simulink model "LUT_kidney_35"  (R2023b)
settings: Solver=FixedStepAuto  StartTime=0  StopTime=10.1  FixedStep=Timegap  RelTol=1e-3
model workspace (MAT data in the model file):
  T1_input = 1.34
(part 2 of 3)

== system LUT_kidney_35/If Action Subsystem6/If Action Subsystem1/If Action Subsystem6/If Action Subsystem4 ==
  In1 : Inport
  Action Port : ActionPort  ActionPortLabel=elseif( u1 >= 1.035)
  LUT 1.04RR : Lookup_n-D  NumberOfTableDimensions=1  BreakpointsForDimension1=[420.026;533.7792;625.1446;723.0482;821.1572;919.1987;1017.154;1115.036;1212.861;1310.64;1408.383;1506.097;1603.789;1701.461;1799.118;1896.76;1994.389]  Table=[400;500;600;700;800;900;1000;1100;1200;1300;1400;1500;1600;1700;1800;1900;2000]  InternalRulePriority=Speed  RndMeth=Simplest
  Out1 : Outport
  wires:
  In1/1 -> LUT 1.04RR/1
  LUT 1.04RR/1 -> Out1/1

== system LUT_kidney_35/If Action Subsystem6/If Action Subsystem1/If Action Subsystem6/If Action Subsystem5 ==
  In1 : Inport
  Action Port : ActionPort  ActionPortLabel=elseif( u1 >= 1.055)
  LUT 1.06RR : Lookup_n-D  NumberOfTableDimensions=1  BreakpointsForDimension1=[419.5192;532.953;624.0409;721.6063;819.3558;917.0247;1014.599;1112.093;1209.526;1306.909;1404.254;1501.569;1598.859;1696.128;1793.38;1890.617;1987.841]  Table=[400;500;600;700;800;900;1000;1100;1200;1300;1400;1500;1600;1700;1800;1900;2000]  InternalRulePriority=Speed  RndMeth=Simplest
  Out1 : Outport
  wires:
  In1/1 -> LUT 1.06RR/1
  LUT 1.06RR/1 -> Out1/1

== system LUT_kidney_35/If Action Subsystem6/If Action Subsystem1/If Action Subsystem6/If Action Subsystem6 ==
  In1 : Inport
  Action Port : ActionPort  ActionPortLabel=elseif( u1 >= 1.045)
  LUT 1.05RR : Lookup_n-D  NumberOfTableDimensions=1  BreakpointsForDimension1=[419.7703;533.3612;624.5658;722.3181;820.245;918.098;1015.86;1113.547;1211.173;1308.752;1406.294;1503.806;1601.294;1698.763;1796.215;1893.652;1991.077]  Table=[400;500;600;700;800;900;1000;1100;1200;1300;1400;1500;1600;1700;1800;1900;2000]  InternalRulePriority=Speed  RndMeth=Simplest
  Out1 : Outport
  wires:
  In1/1 -> LUT 1.05RR/1
  LUT 1.05RR/1 -> Out1/1

== system LUT_kidney_35/If Action Subsystem6/If Action Subsystem1/If Action Subsystem6/If Action Subsystem7 ==
  In1 : Inport
  Action Port : ActionPort  ActionPortLabel=elseif( u1 >= 1.065)
  LUT 1.07RR : Lookup_n-D  NumberOfTableDimensions=1  BreakpointsForDimension1=[419.2724;532.5542;623.5094;720.9123;818.4888;915.9781;1013.368;1110.676;1207.919;1305.111;1402.264;1499.385;1596.48;1693.555;1790.611;1887.653;1984.68]  Table=[400;500;600;700;800;900;1000;1100;1200;1300;1400;1500;1600;1700;1800;1900;2000]  InternalRulePriority=Speed  RndMeth=Simplest
  Out1 : Outport
  wires:
  In1/1 -> LUT 1.07RR/1
  LUT 1.07RR/1 -> Out1/1

== system LUT_kidney_35/If Action Subsystem6/If Action Subsystem1/If Action Subsystem6/If Action Subsystem8 ==
  In1 : Inport
  Action Port : ActionPort  ActionPortLabel=elseif(u1 >= 1.075)
  LUT 1.08RR : Lookup_n-D  NumberOfTableDimensions=1  BreakpointsForDimension1=[419.0299;532.1644;622.9907;720.2354;817.6431;914.9571;1012.167;1109.292;1206.35;1303.355;1400.32;1497.252;1594.157;1691.041;1787.906;1884.756;1981.592]  Table=[400;500;600;700;800;900;1000;1100;1200;1300;1400;1500;1600;1700;1800;1900;2000]  InternalRulePriority=Speed  RndMeth=Simplest
  Out1 : Outport
  wires:
  In1/1 -> LUT 1.08RR/1
  LUT 1.08RR/1 -> Out1/1

== system LUT_kidney_35/If Action Subsystem6/If Action Subsystem1/If Action Subsystem6/If Action Subsystem9 ==
  In1 : Inport
  Action Port : ActionPort  ActionPortLabel=if(u1 >= 1.085)
  LUT 1.09RR : Lookup_n-D  NumberOfTableDimensions=1  BreakpointsForDimension1=[418.7915;531.7834;622.4844;719.5751;816.8181;913.9608;1010.995;1107.941;1204.818;1301.641;1398.421;1495.168;1591.887;1688.584;1785.262;1881.925;1978.573]  Table=[400;500;600;700;800;900;1000;1100;1200;1300;1400;1500;1600;1700;1800;1900;2000]  InternalRulePriority=Speed  RndMeth=Simplest
  Out1 : Outport
  wires:
  In1/1 -> LUT 1.09RR/1
  LUT 1.09RR/1 -> Out1/1

== system LUT_kidney_35/If Action Subsystem6/If Action Subsystem1/If Action Subsystem7/If Action Subsystem1 ==
  In1 : Inport
  Action Port : ActionPort  ActionPortLabel=elseif( u1 >= 1.215)
  LUT 1.22RR : Lookup_n-D  NumberOfTableDimensions=1  BreakpointsForDimension1=[416.0084;527.5016;616.8602;712.2688;807.6951;902.9352;998.0083;1092.951;1187.794;1282.56;1377.266;1471.925;1566.545;1661.135;1755.698;1850.24;1944.764]  Table=[400;500;600;700;800;900;1000;1100;1200;1300;1400;1500;1600;1700;1800;1900;2000]  InternalRulePriority=Speed  RndMeth=Simplest
  Out1 : Outport
  wires:
  In1/1 -> LUT 1.22RR/1
  LUT 1.22RR/1 -> Out1/1

== system LUT_kidney_35/If Action Subsystem6/If Action Subsystem1/If Action Subsystem7/If Action Subsystem10 ==
  In1 : Inport
  Action Port : ActionPort  ActionPortLabel=elseif( u1 >= 1.205)
  LUT 1.21RR : Lookup_n-D  NumberOfTableDimensions=1  BreakpointsForDimension1=[416.2043;527.7926;617.2379;712.7574;808.3047;903.6723;998.8776;1093.956;1188.937;1283.842;1378.69;1473.49;1568.254;1662.987;1757.695;1852.381;1947.05]  Table=[400;500;600;700;800;900;1000;1100;1200;1300;1400;1500;1600;1700;1800;1900;2000]  InternalRulePriority=Speed  RndMeth=Simplest
  Out1 : Outport
  wires:
  In1/1 -> LUT 1.21RR/1
  LUT 1.21RR/1 -> Out1/1

== system LUT_kidney_35/If Action Subsystem6/If Action Subsystem1/If Action Subsystem7/If Action Subsystem2 ==
  In1 : Inport
  Action Port : ActionPort  ActionPortLabel=else
  LUT 1.20RR : Lookup_n-D  NumberOfTableDimensions=1  BreakpointsForDimension1=[416.403;528.0893;617.6239;713.2569;808.928;904.426;999.7663;1094.983;1190.104;1285.152;1380.143;1475.089;1569.998;1664.878;1759.732;1854.566;1949.383]  Table=[400;500;600;700;800;900;1000;1100;1200;1300;1400;1500;1600;1700;1800;1900;2000]  InternalRulePriority=Speed  RndMeth=Simplest
  Out1 : Outport
  wires:
  In1/1 -> LUT 1.20RR/1
  LUT 1.20RR/1 -> Out1/1

== system LUT_kidney_35/If Action Subsystem6/If Action Subsystem1/If Action Subsystem7/If Action Subsystem3 ==
  In1 : Inport
  Action Port : ActionPort  ActionPortLabel=elseif( u1 >= 1.225)
  LUT 1.23RR : Lookup_n-D  NumberOfTableDimensions=1  BreakpointsForDimension1=[415.8151;527.216;616.4903;711.7908;807.0989;902.2141;997.1578;1091.968;1186.676;1281.305;1375.873;1470.392;1564.872;1659.32;1753.742;1848.142;1942.523]  Table=[400;500;600;700;800;900;1000;1100;1200;1300;1400;1500;1600;1700;1800;1900;2000]  InternalRulePriority=Speed  RndMeth=Simplest
  Out1 : Outport
  wires:
  In1/1 -> LUT 1.23RR/1
  LUT 1.23RR/1 -> Out1/1

== system LUT_kidney_35/If Action Subsystem6/If Action Subsystem1/If Action Subsystem7/If Action Subsystem4 ==
  In1 : Inport
  Action Port : ActionPort  ActionPortLabel=elseif( u1 >= 1.235)
  LUT 1.24RR : Lookup_n-D  NumberOfTableDimensions=1  BreakpointsForDimension1=[415.6243;526.9358;616.128;711.3231;806.5156;901.5086;996.3255;1091.006;1185.581;1280.076;1374.508;1468.89;1563.233;1657.543;1751.826;1846.086;1940.327]  Table=[400;500;600;700;800;900;1000;1100;1200;1300;1400;1500;1600;1700;1800;1900;2000]  InternalRulePriority=Speed  RndMeth=Simplest
  Out1 : Outport
  wires:
  In1/1 -> LUT 1.24RR/1
  LUT 1.24RR/1 -> Out1/1

== system LUT_kidney_35/If Action Subsystem6/If Action Subsystem1/If Action Subsystem7/If Action Subsystem5 ==
  In1 : Inport
  Action Port : ActionPort  ActionPortLabel=elseif( u1 >= 1.255)
  LUT 1.26RR : Lookup_n-D  NumberOfTableDimensions=1  BreakpointsForDimension1=[415.2502;526.3909;615.4257;710.4174;805.3864;900.1427;994.7137;1089.141;1183.459;1277.693;1371.861;1465.978;1560.052;1654.093;1748.106;1842.095;1936.064]  Table=[400;500;600;700;800;900;1000;1100;1200;1300;1400;1500;1600;1700;1800;1900;2000]  InternalRulePriority=Speed  RndMeth=Simplest
  Out1 : Outport
  wires:
  In1/1 -> LUT 1.26RR/1
  LUT 1.26RR/1 -> Out1/1

== system LUT_kidney_35/If Action Subsystem6/If Action Subsystem1/If Action Subsystem7/If Action Subsystem6 ==
  In1 : Inport
  Action Port : ActionPort  ActionPortLabel=elseif( u1 >= 1.245)
  LUT 1.25RR : Lookup_n-D  NumberOfTableDimensions=1  BreakpointsForDimension1=[415.4361;526.6608;615.7732;710.8654;805.9449;900.8182;995.511;1090.064;1184.509;1278.872;1373.171;1467.419;1561.626;1655.8;1749.947;1844.071;1938.175]  Table=[400;500;600;700;800;900;1000;1100;1200;1300;1400;1500;1600;1700;1800;1900;2000]  InternalRulePriority=Speed  RndMeth=Simplest
  Out1 : Outport
  wires:
  In1/1 -> LUT 1.25RR/1
  LUT 1.25RR/1 -> Out1/1

== system LUT_kidney_35/If Action Subsystem6/If Action Subsystem1/If Action Subsystem7/If Action Subsystem7 ==
  In1 : Inport
  Action Port : ActionPort  ActionPortLabel=elseif( u1 >= 1.265)
  LUT 1.27RR : Lookup_n-D  NumberOfTableDimensions=1  BreakpointsForDimension1=[415.0668;526.1258;615.0852;709.9789;804.8399;899.4815;993.9333;1088.238;1182.431;1276.538;1370.578;1464.565;1558.51;1652.42;1746.301;1840.158;1933.995]  Table=[400;500;600;700;800;900;1000;1100;1200;1300;1400;1500;1600;1700;1800;1900;2000]  InternalRulePriority=Speed  RndMeth=Simplest
  Out1 : Outport
  wires:
  In1/1 -> LUT 1.27RR/1
  LUT 1.27RR/1 -> Out1/1

== system LUT_kidney_35/If Action Subsystem6/If Action Subsystem1/If Action Subsystem7/If Action Subsystem8 ==
  In1 : Inport
  Action Port : ActionPort  ActionPortLabel=elseif(u1 >= 1.275)
  LUT 1.28RR : Lookup_n-D  NumberOfTableDimensions=1  BreakpointsForDimension1=[414.8856;525.8655;614.7515;709.5496;804.3049;898.8344;993.1693;1087.354;1181.425;1275.407;1369.321;1463.181;1556.998;1650.779;1744.531;1838.259;1931.966]  Table=[400;500;600;700;800;900;1000;1100;1200;1300;1400;1500;1600;1700;1800;1900;2000]  InternalRulePriority=Speed  RndMeth=Simplest
  Out1 : Outport
  wires:
  In1/1 -> LUT 1.28RR/1
  LUT 1.28RR/1 -> Out1/1

== system LUT_kidney_35/If Action Subsystem6/If Action Subsystem1/If Action Subsystem7/If Action Subsystem9 ==
  In1 : Inport
  Action Port : ActionPort  ActionPortLabel=if(u1 >= 1.285)
  LUT 1.29RR : Lookup_n-D  NumberOfTableDimensions=1  BreakpointsForDimension1=[414.7067;525.6098;614.4245;709.1292;803.7813;898.2008;992.4213;1086.488;1180.439;1274.299;1368.089;1461.825;1555.516;1649.171;1742.796;1836.396;1929.975]  Table=[400;500;600;700;800;900;1000;1100;1200;1300;1400;1500;1600;1700;1800;1900;2000]  InternalRulePriority=Speed  RndMeth=Simplest
  Out1 : Outport
  wires:
  In1/1 -> LUT 1.29RR/1
  LUT 1.29RR/1 -> Out1/1

== system LUT_kidney_35/If Action Subsystem6/If Action Subsystem1/If Action Subsystem8/If Action Subsystem1 ==
  In1 : Inport
  Action Port : ActionPort  ActionPortLabel=elseif( u1 >= 1.315)
  LUT 1.32RR : Lookup_n-D  NumberOfTableDimensions=1  BreakpointsForDimension1=[414.1829;524.8694;613.4816;707.9195;802.2751;896.3784;990.2688;1083.996;1177.598;1271.106;1364.539;1457.913;1551.24;1644.53;1737.787;1831.019;1924.228]  Table=[400;500;600;700;800;900;1000;1100;1200;1300;1400;1500;1600;1700;1800;1900;2000]  InternalRulePriority=Speed  RndMeth=Simplest
  Out1 : Outport
  wires:
  In1/1 -> LUT 1.32RR/1
  LUT 1.32RR/1 -> Out1/1

== system LUT_kidney_35/If Action Subsystem6/If Action Subsystem1/If Action Subsystem8/If Action Subsystem10 ==
  In1 : Inport
  Action Port : ActionPort  ActionPortLabel=elseif( u1 >= 1.305)
  LUT 1.31RR : Lookup_n-D  NumberOfTableDimensions=1  BreakpointsForDimension1=[414.3554;525.1119;613.7897;708.3144;802.7666;896.9732;990.9714;1084.81;1178.526;1272.149;1365.699;1459.191;1552.638;1646.047;1739.425;1832.777;1926.107]  Table=[400;500;600;700;800;900;1000;1100;1200;1300;1400;1500;1600;1700;1800;1900;2000]  InternalRulePriority=Speed  RndMeth=Simplest
  Out1 : Outport
  wires:
  In1/1 -> LUT 1.31RR/1
  LUT 1.31RR/1 -> Out1/1

== system LUT_kidney_35/If Action Subsystem6/If Action Subsystem1/If Action Subsystem8/If Action Subsystem2 ==
  In1 : Inport
  Action Port : ActionPort  ActionPortLabel=else
  LUT 1.30RR : Lookup_n-D  NumberOfTableDimensions=1  BreakpointsForDimension1=[414.53;525.3587;614.1039;708.7176;803.2686;897.5805;991.6888;1085.64;1179.472;1273.213;1366.882;1460.495;1554.063;1647.593;1741.094;1834.569;1928.023]  Table=[400;500;600;700;800;900;1000;1100;1200;1300;1400;1500;1600;1700;1800;1900;2000]  InternalRulePriority=Speed  RndMeth=Simplest
  Out1 : Outport
  wires:
  In1/1 -> LUT 1.30RR/1
  LUT 1.30RR/1 -> Out1/1

== system LUT_kidney_35/If Action Subsystem6/If Action Subsystem1/If Action Subsystem8/If Action Subsystem3 ==
  In1 : Inport
  Action Port : ActionPort  ActionPortLabel=elseif( u1 >= 1.325)
  LUT 1.33RR : Lookup_n-D  NumberOfTableDimensions=1  BreakpointsForDimension1=[414.0125;524.6311;613.1794;707.5326;801.7937;895.7959;989.5805;1083.198;1176.689;1270.083;1363.401;1456.66;1549.87;1643.041;1736.181;1829.293;1922.383]  Table=[400;500;600;700;800;900;1000;1100;1200;1300;1400;1500;1600;1700;1800;1900;2000]  InternalRulePriority=Speed  RndMeth=Simplest
  Out1 : Outport
  wires:
  In1/1 -> LUT 1.33RR/1
  LUT 1.33RR/1 -> Out1/1

== system LUT_kidney_35/If Action Subsystem6/If Action Subsystem1/If Action Subsystem8/If Action Subsystem4 ==
  In1 : Inport
  Action Port : ActionPort  ActionPortLabel=elseif( u1 >= 1.335)
  LUT 1.34RR : Lookup_n-D  NumberOfTableDimensions=1  BreakpointsForDimension1=[413.8441;524.3968;612.8831;707.1536;801.3223;895.2254;988.9063;1082.417;1175.799;1269.081;1362.286;1455.431;1548.526;1641.582;1734.605;1827.601;1920.573]  Table=[400;500;600;700;800;900;1000;1100;1200;1300;1400;1500;1600;1700;1800;1900;2000]  InternalRulePriority=Speed  RndMeth=Simplest
  Out1 : Outport
  wires:
  In1/1 -> LUT 1.34RR/1
  LUT 1.34RR/1 -> Out1/1

== system LUT_kidney_35/If Action Subsystem6/If Action Subsystem1/If Action Subsystem8/If Action Subsystem5 ==
  In1 : Inport
  Action Port : ActionPort  ActionPortLabel=elseif( u1 >= 1.355)
  LUT 1.36RR : Lookup_n-D  NumberOfTableDimensions=1  BreakpointsForDimension1=[413.5131;523.94;612.3074;706.4184;800.4081;894.1191;987.5986;1080.901;1174.07;1267.135;1360.12;1453.043;1545.914;1638.744;1731.541;1824.309;1917.053]  Table=[400;500;600;700;800;900;1000;1100;1200;1300;1400;1500;1600;1700;1800;1900;2000]  InternalRulePriority=Speed  RndMeth=Simplest
  Out1 : Outport
  wires:
  In1/1 -> LUT 1.36RR/1
  LUT 1.36RR/1 -> Out1/1

== system LUT_kidney_35/If Action Subsystem6/If Action Subsystem1/If Action Subsystem8/If Action Subsystem6 ==
  In1 : Inport
  Action Port : ActionPort  ActionPortLabel=elseif( u1 >= 1.345)
  LUT 1.35RR : Lookup_n-D  NumberOfTableDimensions=1  BreakpointsForDimension1=[413.6776;524.1665;612.5925;706.7823;800.8605;894.6666;988.2458;1081.652;1174.926;1268.098;1361.193;1454.225;1547.207;1640.149;1733.058;1825.939;1918.797]  Table=[400;500;600;700;800;900;1000;1100;1200;1300;1400;1500;1600;1700;1800;1900;2000]  InternalRulePriority=Speed  RndMeth=Simplest
  Out1 : Outport
  wires:
  In1/1 -> LUT 1.35RR/1
  LUT 1.35RR/1 -> Out1/1

== system LUT_kidney_35/If Action Subsystem6/If Action Subsystem1/If Action Subsystem8/If Action Subsystem7 ==
  In1 : Inport
  Action Port : ActionPort  ActionPortLabel=elseif( u1 >= 1.365)
  LUT 1.37RR : Lookup_n-D  NumberOfTableDimensions=1  BreakpointsForDimension1=[413.3504;523.7173;612.0277;706.0618;799.9648;893.5827;986.9645;1080.166;1173.231;1266.19;1359.069;1451.883;1544.645;1637.365;1730.051;1822.708;1915.341]  Table=[400;500;600;700;800;900;1000;1100;1200;1300;1400;1500;1600;1700;1800;1900;2000]  InternalRulePriority=Speed  RndMeth=Simplest
  Out1 : Outport
  wires:
  In1/1 -> LUT 1.37RR/1
  LUT 1.37RR/1 -> Out1/1

== system LUT_kidney_35/If Action Subsystem6/If Action Subsystem1/If Action Subsystem8/If Action Subsystem8 ==
  In1 : Inport
  Action Port : ActionPort  ActionPortLabel=elseif(u1 >= 1.375)
  LUT 1.38RR : Lookup_n-D  NumberOfTableDimensions=1  BreakpointsForDimension1=[413.1896;523.4982;611.7533;705.7122;799.5306;893.0572;986.343;1079.445;1172.408;1265.264;1358.037;1450.745;1543.399;1636.012;1728.589;1821.137;1913.66]  Table=[400;500;600;700;800;900;1000;1100;1200;1300;1400;1500;1600;1700;1800;1900;2000]  InternalRulePriority=Speed  RndMeth=Simplest
  Out1 : Outport
  wires:
  In1/1 -> LUT 1.38RR/1
  LUT 1.38RR/1 -> Out1/1

== system LUT_kidney_35/If Action Subsystem6/If Action Subsystem1/If Action Subsystem8/If Action Subsystem9 ==
  In1 : Inport
  Action Port : ActionPort  ActionPortLabel=if(u1 >= 1.385)
  LUT 1.39RR : Lookup_n-D  NumberOfTableDimensions=1  BreakpointsForDimension1=[413.0306;523.2827;611.4839;705.3696;799.1051;892.5422;985.7339;1078.739;1171.601;1264.356;1357.025;1449.628;1542.177;1634.683;1727.154;1819.594;1912.01]  Table=[400;500;600;700;800;900;1000;1100;1200;1300;1400;1500;1600;1700;1800;1900;2000]  InternalRulePriority=Speed  RndMeth=Simplest
  Out1 : Outport
  wires:
  In1/1 -> LUT 1.39RR/1
  LUT 1.39RR/1 -> Out1/1

== system LUT_kidney_35/If Action Subsystem6/If Action Subsystem1/If Action Subsystem9/If Action Subsystem1 ==
  In1 : Inport
  Action Port : ActionPort  ActionPortLabel=elseif( u1 >= 1.415)
  LUT 1.42RR : Lookup_n-D  NumberOfTableDimensions=1  BreakpointsForDimension1=[412.5639;522.6569;610.7055;704.3815;797.8789;891.0583;983.9782;1076.701;1169.274;1261.733;1354.103;1446.402;1538.645;1630.843;1723.003;1815.131;1907.234]  Table=[400;500;600;700;800;900;1000;1100;1200;1300;1400;1500;1600;1700;1800;1900;2000]  InternalRulePriority=Speed  RndMeth=Simplest
  Out1 : Outport
  wires:
  In1/1 -> LUT 1.42RR/1
  LUT 1.42RR/1 -> Out1/1

== system LUT_kidney_35/If Action Subsystem6/If Action Subsystem1/If Action Subsystem9/If Action Subsystem10 ==
  In1 : Inport
  Action Port : ActionPort  ActionPortLabel=elseif( u1 >= 1.405)
  LUT 1.41RR : Lookup_n-D  NumberOfTableDimensions=1  BreakpointsForDimension1=[412.7178;522.8621;610.9602;704.7044;798.2794;891.543;984.5518;1077.367;1170.035;1262.59;1355.058;1447.457;1539.801;1632.099;1724.361;1816.592;1908.797]  Table=[400;500;600;700;800;900;1000;1100;1200;1300;1400;1500;1600;1700;1800;1900;2000]  InternalRulePriority=Speed  RndMeth=Simplest
  Out1 : Outport
  wires:
  In1/1 -> LUT 1.41RR/1
  LUT 1.41RR/1 -> Out1/1

== system LUT_kidney_35/If Action Subsystem6/If Action Subsystem1/If Action Subsystem9/If Action Subsystem2 ==
  In1 : Inport
  Action Port : ActionPort  ActionPortLabel=else
  LUT 1.40RR : Lookup_n-D  NumberOfTableDimensions=1  BreakpointsForDimension1=[412.8733;523.0707;611.2196;705.0337;798.6881;892.0376;985.137;1078.046;1170.81;1263.464;1356.032;1448.532;1540.978;1633.38;1725.745;1818.08;1910.389]  Table=[400;500;600;700;800;900;1000;1100;1200;1300;1400;1500;1600;1700;1800;1900;2000]  InternalRulePriority=Speed  RndMeth=Simplest
  Out1 : Outport
  wires:
  In1/1 -> LUT 1.40RR/1
  LUT 1.40RR/1 -> Out1/1

== system LUT_kidney_35/If Action Subsystem6/If Action Subsystem1/If Action Subsystem9/If Action Subsystem3 ==
  In1 : Inport
  Action Port : ActionPort  ActionPortLabel=elseif( u1 >= 1.425)
  LUT 1.43RR : Lookup_n-D  NumberOfTableDimensions=1  BreakpointsForDimension1=[412.4118;522.4548;610.4555;704.0649;797.4863;890.5831;983.4159;1076.048;1168.528;1260.892;1353.165;1445.366;1537.511;1629.609;1721.669;1813.697;1905.698]  Table=[400;500;600;700;800;900;1000;1100;1200;1300;1400;1500;1600;1700;1800;1900;2000]  InternalRulePriority=Speed  RndMeth=Simplest
  Out1 : Outport
  wires:
  In1/1 -> LUT 1.43RR/1
  LUT 1.43RR/1 -> Out1/1

== system LUT_kidney_35/If Action Subsystem6/If Action Subsystem1/If Action Subsystem9/If Action Subsystem4 ==
  In1 : Inport
  Action Port : ActionPort  ActionPortLabel=elseif( u1 >= 1.435)
  LUT 1.44RR : Lookup_n-D  NumberOfTableDimensions=1  BreakpointsForDimension1=[412.2612;522.256;610.21;703.7545;797.1014;890.1174;982.8646;1075.408;1167.796;1260.066;1352.244;1444.35;1536.397;1628.397;1720.359;1812.288;1904.189]  Table=[400;500;600;700;800;900;1000;1100;1200;1300;1400;1500;1600;1700;1800;1900;2000]  InternalRulePriority=Speed  RndMeth=Simplest
  Out1 : Outport
  wires:
  In1/1 -> LUT 1.44RR/1
  LUT 1.44RR/1 -> Out1/1

== system LUT_kidney_35/If Action Subsystem6/If Action Subsystem1/If Action Subsystem9/If Action Subsystem5 ==
  In1 : Inport
  Action Port : ActionPort  ActionPortLabel=elseif( u1 >= 1.455)
  LUT 1.46RR : Lookup_n-D  NumberOfTableDimensions=1  BreakpointsForDimension1=[411.965;521.8675;609.7322;703.1513;796.3542;889.2132;981.794;1074.164;1166.374;1258.462;1350.455;1442.372;1534.23;1626.039;1717.808;1809.543;1901.251]  Table=[400;500;600;700;800;900;1000;1100;1200;1300;1400;1500;1600;1700;1800;1900;2000]  InternalRulePriority=Speed  RndMeth=Simplest
  Out1 : Outport
  wires:
  In1/1 -> LUT 1.46RR/1
  LUT 1.46RR/1 -> Out1/1

== system LUT_kidney_35/If Action Subsystem6/If Action Subsystem1/If Action Subsystem9/If Action Subsystem6 ==
  In1 : Inport
  Action Port : ActionPort  ActionPortLabel=elseif( u1 >= 1.445)
  LUT 1.45RR : Lookup_n-D  NumberOfTableDimensions=1  BreakpointsForDimension1=[412.1123;522.0602;609.9689;703.45;796.7241;889.6608;982.324;1074.78;1167.078;1259.256;1351.341;1443.352;1535.304;1627.207;1719.072;1810.903;1902.707]  Table=[400;500;600;700;800;900;1000;1100;1200;1300;1400;1500;1600;1700;1800;1900;2000]  InternalRulePriority=Speed  RndMeth=Simplest
  Out1 : Outport
  wires:
  In1/1 -> LUT 1.45RR/1
  LUT 1.45RR/1 -> Out1/1

== system LUT_kidney_35/If Action Subsystem6/If Action Subsystem1/If Action Subsystem9/If Action Subsystem7 ==
  In1 : Inport
  Action Port : ActionPort  ActionPortLabel=elseif( u1 >= 1.465)
  LUT 1.47RR : Lookup_n-D  NumberOfTableDimensions=1  BreakpointsForDimension1=[411.8192;521.6777;609.4996;702.8584;795.9916;888.7743;981.2742;1073.56;1165.683;1257.682;1349.584;1441.411;1533.176;1624.891;1716.566;1808.207;1899.82]  Table=[400;500;600;700;800;900;1000;1100;1200;1300;1400;1500;1600;1700;1800;1900;2000]  InternalRulePriority=Speed  RndMeth=Simplest
  Out1 : Outport
  wires:
  In1/1 -> LUT 1.47RR/1
  LUT 1.47RR/1 -> Out1/1

== system LUT_kidney_35/If Action Subsystem6/If Action Subsystem1/If Action Subsystem9/If Action Subsystem8 ==
  In1 : Inport
  Action Port : ActionPort  ActionPortLabel=elseif(u1 >= 1.475)
  LUT 1.48RR : Lookup_n-D  NumberOfTableDimensions=1  BreakpointsForDimension1=[411.6749;521.4908;609.2713;702.571;795.636;888.344;980.7645;1072.967;1165.005;1256.917;1348.73;1440.466;1532.14;1623.764;1715.346;1806.894;1898.413]  Table=[400;500;600;700;800;900;1000;1100;1200;1300;1400;1500;1600;1700;1800;1900;2000]  InternalRulePriority=Speed  RndMeth=Simplest
  Out1 : Outport
  wires:
  In1/1 -> LUT 1.48RR/1
  LUT 1.48RR/1 -> Out1/1

== system LUT_kidney_35/If Action Subsystem6/If Action Subsystem1/If Action Subsystem9/If Action Subsystem9 ==
  In1 : Inport
  Action Port : ActionPort  ActionPortLabel=if(u1 >= 1.485)
  LUT 1.49RR : Lookup_n-D  NumberOfTableDimensions=1  BreakpointsForDimension1=[411.5321;521.3067;609.0469;702.2891;795.2873;887.922;980.2646;1072.386;1164.34;1256.165;1347.891;1439.539;1531.123;1622.656;1714.148;1805.604;1897.031]  Table=[400;500;600;700;800;900;1000;1100;1200;1300;1400;1500;1600;1700;1800;1900;2000]  InternalRulePriority=Speed  RndMeth=Simplest
  Out1 : Outport
  wires:
  In1/1 -> LUT 1.49RR/1
  LUT 1.49RR/1 -> Out1/1

== system LUT_kidney_35/If Action Subsystem6/If Action Subsystem2/If Action Subsystem5/If Action Subsystem1 ==
  In1 : Inport
  Action Port : ActionPort  ActionPortLabel=elseif( u1 >= 1.615)
  LUT 1.62RR : Lookup_n-D  NumberOfTableDimensions=1  BreakpointsForDimension1=[409.8015;519.1447;606.459;699.0681;791.3171;883.1195;974.569;1065.752;1156.734;1247.561;1338.268;1428.88;1519.417;1609.892;1700.316;1790.698;1881.045]  Table=[400;500;600;700;800;900;1000;1100;1200;1300;1400;1500;1600;1700;1800;1900;2000]  InternalRulePriority=Speed  RndMeth=Simplest
  Out1 : Outport
  wires:
  In1/1 -> LUT 1.62RR/1
  LUT 1.62RR/1 -> Out1/1

== system LUT_kidney_35/If Action Subsystem6/If Action Subsystem2/If Action Subsystem5/If Action Subsystem10 ==
  In1 : Inport
  Action Port : ActionPort  ActionPortLabel=elseif( u1>= 1.605)
  LUT 1.61RR : Lookup_n-D  NumberOfTableDimensions=1  BreakpointsForDimension1=[409.9269;519.2971;606.6384;699.2892;791.5887;883.4479;974.9589;1066.207;1157.256;1248.153;1338.931;1429.616;1520.226;1610.775;1701.275;1791.733;1882.156]  Table=[400;500;600;700;800;900;1000;1100;1200;1300;1400;1500;1600;1700;1800;1900;2000]  InternalRulePriority=Speed  RndMeth=Simplest
  Out1 : Outport
  wires:
  In1/1 -> LUT 1.61RR/1
  LUT 1.61RR/1 -> Out1/1

== system LUT_kidney_35/If Action Subsystem6/If Action Subsystem2/If Action Subsystem5/If Action Subsystem2 ==
  In1 : Inport
  Action Port : ActionPort  ActionPortLabel=else
  LUT 1.60RR : Lookup_n-D  NumberOfTableDimensions=1  BreakpointsForDimension1=[410.0535;519.4517;606.8208;699.5145;791.8656;883.7827;975.3562;1066.67;1157.788;1248.756;1339.606;1430.365;1521.05;1611.674;1702.25;1792.784;1883.285]  Table=[400;500;600;700;800;900;1000;1100;1200;1300;1400;1500;1600;1700;1800;1900;2000]  InternalRulePriority=Speed  RndMeth=Simplest
  Out1 : Outport
  wires:
  In1/1 -> LUT 1.60RR/1
  LUT 1.60RR/1 -> Out1/1

== system LUT_kidney_35/If Action Subsystem6/If Action Subsystem2/If Action Subsystem5/If Action Subsystem3 ==
  In1 : Inport
  Action Port : ActionPort  ActionPortLabel=elseif( u1 >= 1.625)
  LUT 1.63RR : Lookup_n-D  NumberOfTableDimensions=1  BreakpointsForDimension1=[409.6773;518.9944;606.2826;698.8509;791.0505;882.7972;974.1864;1065.306;1156.221;1246.979;1337.616;1428.157;1518.621;1609.023;1699.373;1789.681;1879.953]  Table=[400;500;600;700;800;900;1000;1100;1200;1300;1400;1500;1600;1700;1800;1900;2000]  InternalRulePriority=Speed  RndMeth=Simplest
  Out1 : Outport
  wires:
  In1/1 -> LUT 1.63RR/1
  LUT 1.63RR/1 -> Out1/1

== system LUT_kidney_35/If Action Subsystem6/If Action Subsystem2/If Action Subsystem5/If Action Subsystem4 ==
  In1 : Inport
  Action Port : ActionPort  ActionPortLabel=elseif( u1 >= 1.635)
  LUT 1.64RR : Lookup_n-D  NumberOfTableDimensions=1  BreakpointsForDimension1=[409.5542;518.8461;606.1091;698.6376;790.7889;882.4803;973.8109;1064.867;1155.717;1246.408;1336.976;1427.446;1517.839;1608.168;1698.446;1788.68;1878.879]  Table=[400;500;600;700;800;900;1000;1100;1200;1300;1400;1500;1600;1700;1800;1900;2000]  InternalRulePriority=Speed  RndMeth=Simplest
  Out1 : Outport
  wires:
  In1/1 -> LUT 1.64RR/1
  LUT 1.64RR/1 -> Out1/1

== system LUT_kidney_35/If Action Subsystem6/If Action Subsystem2/If Action Subsystem5/If Action Subsystem5 ==
  In1 : Inport
  Action Port : ActionPort  ActionPortLabel=elseif( u1 >= 1.655)
  LUT 1.66RR : Lookup_n-D  NumberOfTableDimensions=1  BreakpointsForDimension1=[409.3117;518.5555;605.7705;698.2225;790.2803;881.8663;973.0807;1064.015;1154.736;1245.296;1335.729;1426.061;1516.314;1606.502;1696.637;1786.728;1876.781]  Table=[400;500;600;700;800;900;1000;1100;1200;1300;1400;1500;1600;1700;1800;1900;2000]  InternalRulePriority=Speed  RndMeth=Simplest
  Out1 : Outport
  wires:
  In1/1 -> LUT 1.66RR/1
  LUT 1.66RR/1 -> Out1/1

== system LUT_kidney_35/If Action Subsystem6/If Action Subsystem2/If Action Subsystem5/If Action Subsystem6 ==
  In1 : Inport
  Action Port : ActionPort  ActionPortLabel=elseif( u1 >= 1.645)
  LUT 1.65RR : Lookup_n-D  NumberOfTableDimensions=1  BreakpointsForDimension1=[409.4324;518.6998;605.9384;698.4282;790.5322;882.1708;973.4424;1064.437;1155.222;1245.847;1336.347;1426.748;1517.07;1607.328;1697.534;1787.696;1877.821]  Table=[400;500;600;700;800;900;1000;1100;1200;1300;1400;1500;1600;1700;1800;1900;2000]  InternalRulePriority=Speed  RndMeth=Simplest
  Out1 : Outport
  wires:
  In1/1 -> LUT 1.65RR/1
  LUT 1.65RR/1 -> Out1/1

== system LUT_kidney_35/If Action Subsystem6/If Action Subsystem2/If Action Subsystem5/If Action Subsystem7 ==
  In1 : Inport
  Action Port : ActionPort  ActionPortLabel=elseif( u1 >= 1.665)
  LUT 1.67RR : Lookup_n-D  NumberOfTableDimensions=1  BreakpointsForDimension1=[409.1921;518.4132;605.6053;698.0205;790.033;881.5675;972.7257;1063.6;1154.259;1244.754;1335.121;1425.387;1515.571;1605.69;1695.755;1785.775;1875.758]  Table=[400;500;600;700;800;900;1000;1100;1200;1300;1400;1500;1600;1700;1800;1900;2000]  InternalRulePriority=Speed  RndMeth=Simplest
  Out1 : Outport
  wires:
  In1/1 -> LUT 1.67RR/1
  LUT 1.67RR/1 -> Out1/1

== system LUT_kidney_35/If Action Subsystem6/If Action Subsystem2/If Action Subsystem5/If Action Subsystem8 ==
  In1 : Inport
  Action Port : ActionPort  ActionPortLabel=elseif(u1 >= 1.675)
  LUT 1.68RR : Lookup_n-D  NumberOfTableDimensions=1  BreakpointsForDimension1=[409.0736;518.2727;605.4428;697.8221;789.7904;881.2743;972.3773;1063.193;1153.791;1244.222;1334.524;1424.723;1514.841;1604.891;1694.887;1784.838;1874.751]  Table=[400;500;600;700;800;900;1000;1100;1200;1300;1400;1500;1600;1700;1800;1900;2000]  InternalRulePriority=Speed  RndMeth=Simplest
  Out1 : Outport
  wires:
  In1/1 -> LUT 1.68RR/1
  LUT 1.68RR/1 -> Out1/1

== system LUT_kidney_35/If Action Subsystem6/If Action Subsystem2/If Action Subsystem5/If Action Subsystem9 ==
  In1 : Inport
  Action Port : ActionPort  ActionPortLabel=if(u1 >= 1.685)
  LUT 1.69RR : Lookup_n-D  NumberOfTableDimensions=1  BreakpointsForDimension1=[408.9562;518.1341;605.2828;697.6273;789.5522;880.9866;972.0354;1062.793;1153.331;1243.7;1333.938;1424.071;1514.122;1604.106;1694.034;1783.916;1873.759]  Table=[400;500;600;700;800;900;1000;1100;1200;1300;1400;1500;1600;1700;1800;1900;2000]  InternalRulePriority=Speed  RndMeth=Simplest
  Out1 : Outport
  wires:
  In1/1 -> LUT 1.69RR/1
  LUT 1.69RR/1 -> Out1/1

== system LUT_kidney_35/If Action Subsystem6/If Action Subsystem2/If Action Subsystem6/If Action Subsystem1 ==
  In1 : Inport
  Action Port : ActionPort  ActionPortLabel=elseif( u1 >= 1.515)
  LUT 1.52RR : Lookup_n-D  NumberOfTableDimensions=1  BreakpointsForDimension1=[411.1125;520.7708;608.3971;701.4748;794.281;886.7045;978.8217;1070.707;1162.418;1253.994;1345.466;1436.855;1528.179;1619.449;1710.676;1801.866;1893.025]  Table=[400;500;600;700;800;900;1000;1100;1200;1300;1400;1500;1600;1700;1800;1900;2000]  InternalRulePriority=Speed  RndMeth=Simplest
  Out1 : Outport
  wires:
  In1/1 -> LUT 1.52RR/1
  LUT 1.52RR/1 -> Out1/1

== system LUT_kidney_35/If Action Subsystem6/If Action Subsystem2/If Action Subsystem6/If Action Subsystem10 ==
  In1 : Inport
  Action Port : ActionPort  ActionPortLabel=elseif( u1 >= 1.505)
  LUT 1.51RR : Lookup_n-D  NumberOfTableDimensions=1  BreakpointsForDimension1=[411.2509;520.9468;608.6099;701.7411;794.6099;887.1024;979.2934;1071.256;1163.046;1254.704;1346.26;1437.734;1529.143;1620.5;1711.813;1803.09;1894.337]  Table=[400;500;600;700;800;900;1000;1100;1200;1300;1400;1500;1600;1700;1800;1900;2000]  InternalRulePriority=Speed  RndMeth=Simplest
  Out1 : Outport
  wires:
  In1/1 -> LUT 1.51RR/1
  LUT 1.51RR/1 -> Out1/1

== system LUT_kidney_35/If Action Subsystem6/If Action Subsystem2/If Action Subsystem6/If Action Subsystem2 ==
  In1 : Inport
  Action Port : ActionPort  ActionPortLabel=else
  LUT 1.50RR : Lookup_n-D  NumberOfTableDimensions=1  BreakpointsForDimension1=[411.3908;521.1254;608.8265;702.0125;794.9453;887.5082;979.7743;1071.816;1163.687;1255.428;1347.068;1438.628;1530.124;1621.568;1712.97;1804.336;1895.673]  Table=[400;500;600;700;800;900;1000;1100;1200;1300;1400;1500;1600;1700;1800;1900;2000]  InternalRulePriority=Speed  RndMeth=Simplest
  Out1 : Outport
  wires:
  In1/1 -> LUT 1.50RR/1
  LUT 1.50RR/1 -> Out1/1

== system LUT_kidney_35/If Action Subsystem6/If Action Subsystem2/If Action Subsystem6/If Action Subsystem3 ==
  In1 : Inport
  Action Port : ActionPort  ActionPortLabel=elseif( u1 >= 1.525)
  LUT 1.53RR : Lookup_n-D  NumberOfTableDimensions=1  BreakpointsForDimension1=[410.9755;520.5974;608.188;701.2134;793.9584;886.3141;978.359;1070.169;1161.801;1253.296;1344.686;1435.993;1527.232;1618.417;1709.558;1800.662;1891.734]  Table=[400;500;600;700;800;900;1000;1100;1200;1300;1400;1500;1600;1700;1800;1900;2000]  InternalRulePriority=Speed  RndMeth=Simplest
  Out1 : Outport
  wires:
  In1/1 -> LUT 1.53RR/1
  LUT 1.53RR/1 -> Out1/1

== system LUT_kidney_35/If Action Subsystem6/If Action Subsystem2/If Action Subsystem6/If Action Subsystem4 ==
  In1 : Inport
  Action Port : ActionPort  ActionPortLabel=elseif( u1 >= 1.535)
  LUT 1.54RR : Lookup_n-D  NumberOfTableDimensions=1  BreakpointsForDimension1=[410.8398;520.4266;607.9825;700.957;793.642;885.9313;977.9051;1069.64;1161.195;1252.612;1343.921;1435.145;1526.302;1617.403;1708.46;1799.478;1890.465]  Table=[400;500;600;700;800;900;1000;1100;1200;1300;1400;1500;1600;1700;1800;1900;2000]  InternalRulePriority=Speed  RndMeth=Simplest
  Out1 : Outport
  wires:
  In1/1 -> LUT 1.54RR/1
  LUT 1.54RR/1 -> Out1/1

== system LUT_kidney_35/If Action Subsystem6/If Action Subsystem2/If Action Subsystem6/If Action Subsystem5 ==
  In1 : Inport
  Action Port : ActionPort  ActionPortLabel=elseif( u1 >= 1.555)
  LUT 1.56RR : Lookup_n-D  NumberOfTableDimensions=1  BreakpointsForDimension1=[410.5725;520.0923;607.582;700.4582;793.027;885.1874;977.0229;1068.613;1160.017;1251.279;1342.431;1433.495;1524.49;1615.427;1706.319;1797.171;1887.991]  Table=[400;500;600;700;800;900;1000;1100;1200;1300;1400;1500;1600;1700;1800;1900;2000]  InternalRulePriority=Speed  RndMeth=Simplest
  Out1 : Outport
  wires:
  In1/1 -> LUT 1.56RR/1
  LUT 1.56RR/1 -> Out1/1

== system LUT_kidney_35/If Action Subsystem6/If Action Subsystem2/If Action Subsystem6/If Action Subsystem6 ==
  In1 : Inport
  Action Port : ActionPort  ActionPortLabel=elseif( u1 >= 1.545)
  LUT 1.55RR : Lookup_n-D  NumberOfTableDimensions=1  BreakpointsForDimension1=[410.7055;520.2582;607.7805;700.7053;793.3316;885.5558;977.4598;1069.122;1160.601;1251.939;1343.169;1434.313;1525.388;1616.407;1707.38;1798.315;1889.218]  Table=[400;500;600;700;800;900;1000;1100;1200;1300;1400;1500;1600;1700;1800;1900;2000]  InternalRulePriority=Speed  RndMeth=Simplest
  Out1 : Outport
  wires:
  In1/1 -> LUT 1.55RR/1
  LUT 1.55RR/1 -> Out1/1

== system LUT_kidney_35/If Action Subsystem6/If Action Subsystem2/If Action Subsystem6/If Action Subsystem7 ==
  In1 : Inport
  Action Port : ActionPort  ActionPortLabel=elseif( u1 >= 1.565)
  LUT 1.57RR : Lookup_n-D  NumberOfTableDimensions=1  BreakpointsForDimension1=[410.4408;519.9287;607.3868;700.2157;792.7283;884.8261;976.5943;1068.114;1159.444;1250.631;1341.706;1432.692;1523.607;1614.465;1705.275;1796.047;1886.785]  Table=[400;500;600;700;800;900;1000;1100;1200;1300;1400;1500;1600;1700;1800;1900;2000]  InternalRulePriority=Speed  RndMeth=Simplest
  Out1 : Outport
  wires:
  In1/1 -> LUT 1.57RR/1
  LUT 1.57RR/1 -> Out1/1

== system LUT_kidney_35/If Action Subsystem6/If Action Subsystem2/If Action Subsystem6/If Action Subsystem8 ==
  In1 : Inport
  Action Port : ActionPort  ActionPortLabel=elseif(u1 >= 1.575)
  LUT 1.58RR : Lookup_n-D  NumberOfTableDimensions=1  BreakpointsForDimension1=[410.3104;519.7674;607.195;699.9776;792.4352;884.4716;976.1738;1067.623;1158.882;1249.995;1340.993;1431.902;1522.74;1613.519;1704.25;1794.941;1885.599]  Table=[400;500;600;700;800;900;1000;1100;1200;1300;1400;1500;1600;1700;1800;1900;2000]  InternalRulePriority=Speed  RndMeth=Simplest
  Out1 : Outport
  wires:
  In1/1 -> LUT 1.58RR/1
  LUT 1.58RR/1 -> Out1/1

== system LUT_kidney_35/If Action Subsystem6/If Action Subsystem2/If Action Subsystem6/If Action Subsystem9 ==
  In1 : Inport
  Action Port : ActionPort  ActionPortLabel=if(u1 >= 1.585)
  LUT 1.59RR : Lookup_n-D  NumberOfTableDimensions=1  BreakpointsForDimension1=[410.1813;519.6085;607.0063;699.7439;792.1477;884.1239;975.7611;1067.142;1158.33;1249.37;1340.294;1431.127;1521.887;1612.588;1703.241;1793.854;1884.432]  Table=[400;500;600;700;800;900;1000;1100;1200;1300;1400;1500;1600;1700;1800;1900;2000]  InternalRulePriority=Speed  RndMeth=Simplest
  Out1 : Outport
  wires:
  In1/1 -> LUT 1.59RR/1
  LUT 1.59RR/1 -> Out1/1

== system LUT_kidney_35/If Action Subsystem6/If Action Subsystem2/If Action Subsystem7/If Action Subsystem1 ==
  In1 : Inport
  Action Port : ActionPort  ActionPortLabel=elseif( u1 >= 1.715)
  LUT 1.72RR : Lookup_n-D  NumberOfTableDimensions=1  BreakpointsForDimension1=[408.6106;517.7291;604.8183;697.0631;788.8636;880.155;971.0469;1061.637;1152;1242.187;1332.238;1422.181;1512.038;1601.825;1691.555;1781.237;1870.879]  Table=[400;500;600;700;800;900;1000;1100;1200;1300;1400;1500;1600;1700;1800;1900;2000]  InternalRulePriority=Speed  RndMeth=Simplest
  Out1 : Outport
  wires:
  In1/1 -> LUT 1.72RR/1
  LUT 1.72RR/1 -> Out1/1

== system LUT_kidney_35/If Action Subsystem6/If Action Subsystem2/If Action Subsystem7/If Action Subsystem10 ==
  In1 : Inport
  Action Port : ActionPort  ActionPortLabel=elseif( u1>= 1.705)
  LUT 1.71RR : Lookup_n-D  NumberOfTableDimensions=1  BreakpointsForDimension1=[408.7247;517.8623;604.9707;697.2478;789.0889;880.427;971.3703;1062.016;1152.435;1242.682;1332.794;1422.8;1512.721;1602.573;1692.368;1782.116;1871.824]  Table=[400;500;600;700;800;900;1000;1100;1200;1300;1400;1500;1600;1700;1800;1900;2000]  InternalRulePriority=Speed  RndMeth=Simplest
  Out1 : Outport
  wires:
  In1/1 -> LUT 1.71RR/1
  LUT 1.71RR/1 -> Out1/1

== system LUT_kidney_35/If Action Subsystem6/If Action Subsystem2/If Action Subsystem7/If Action Subsystem2 ==
  In1 : Inport
  Action Port : ActionPort  ActionPortLabel=else
  LUT 1.70RR : Lookup_n-D  NumberOfTableDimensions=1  BreakpointsForDimension1=[408.84;517.9973;605.1255;697.4359;789.3184;880.7042;971.6997;1062.401;1152.879;1243.187;1333.361;1423.431;1513.416;1603.333;1693.194;1783.009;1872.784]  Table=[400;500;600;700;800;900;1000;1100;1200;1300;1400;1500;1600;1700;1800;1900;2000]  InternalRulePriority=Speed  RndMeth=Simplest
  Out1 : Outport
  wires:
  In1/1 -> LUT 1.70RR/1
  LUT 1.70RR/1 -> Out1/1

== system LUT_kidney_35/If Action Subsystem6/If Action Subsystem2/If Action Subsystem7/If Action Subsystem3 ==
  In1 : Inport
  Action Port : ActionPort  ActionPortLabel=elseif( u1 >= 1.725)
  LUT 1.73RR : Lookup_n-D  NumberOfTableDimensions=1  BreakpointsForDimension1=[408.4975;517.5976;604.6683;696.8817;788.6425;879.8881;970.7295;1061.266;1151.571;1241.7;1331.69;1421.572;1511.367;1601.09;1690.756;1780.373;1869.95]  Table=[400;500;600;700;800;900;1000;1100;1200;1300;1400;1500;1600;1700;1800;1900;2000]  InternalRulePriority=Speed  RndMeth=Simplest
  Out1 : Outport
  wires:
  In1/1 -> LUT 1.73RR/1
  LUT 1.73RR/1 -> Out1/1

== system LUT_kidney_35/If Action Subsystem6/If Action Subsystem2/If Action Subsystem7/If Action Subsystem4 ==
  In1 : Inport
  Action Port : ActionPort  ActionPortLabel=elseif( u1 >= 1.735)
  LUT 1.74RR : Lookup_n-D  NumberOfTableDimensions=1  BreakpointsForDimension1=[408.3854;517.4678;604.5207;696.7034;788.4255;879.6261;970.4179;1060.901;1151.151;1241.222;1331.153;1420.973;1510.706;1600.367;1689.969;1779.522;1869.034]  Table=[400;500;600;700;800;900;1000;1100;1200;1300;1400;1500;1600;1700;1800;1900;2000]  InternalRulePriority=Speed  RndMeth=Simplest
  Out1 : Outport
  wires:
  In1/1 -> LUT 1.74RR/1
  LUT 1.74RR/1 -> Out1/1

== system LUT_kidney_35/If Action Subsystem6/If Action Subsystem2/If Action Subsystem7/If Action Subsystem5 ==
  In1 : Inport
  Action Port : ActionPort  ActionPortLabel=elseif( u1 >= 1.755)
  LUT 1.76RR : Lookup_n-D  NumberOfTableDimensions=1  BreakpointsForDimension1=[408.1643;517.2131;604.2323;696.3562;788.0032;879.1166;969.8119;1060.192;1150.332;1240.29;1330.104;1419.806;1509.417;1598.955;1688.433;1777.861;1867.246]  Table=[400;500;600;700;800;900;1000;1100;1200;1300;1400;1500;1600;1700;1800;1900;2000]  InternalRulePriority=Speed  RndMeth=Simplest
  Out1 : Outport
  wires:
  In1/1 -> LUT 1.76RR/1
  LUT 1.76RR/1 -> Out1/1

== system LUT_kidney_35/If Action Subsystem6/If Action Subsystem2/If Action Subsystem7/If Action Subsystem6 ==
  In1 : Inport
  Action Port : ActionPort  ActionPortLabel=elseif( u1 >= 1.745)
  LUT 1.75RR : Lookup_n-D  NumberOfTableDimensions=1  BreakpointsForDimension1=[408.2743;517.3396;604.3754;696.5283;788.2124;879.369;970.1121;1060.543;1150.738;1240.752;1330.624;1420.385;1510.056;1599.655;1689.195;1778.685;1868.133]  Table=[400;500;600;700;800;900;1000;1100;1200;1300;1400;1500;1600;1700;1800;1900;2000]  InternalRulePriority=Speed  RndMeth=Simplest
  Out1 : Outport
  wires:
  In1/1 -> LUT 1.75RR/1
  LUT 1.75RR/1 -> Out1/1

== system LUT_kidney_35/If Action Subsystem6/If Action Subsystem2/If Action Subsystem7/If Action Subsystem7 ==
  In1 : Inport
  Action Port : ActionPort  ActionPortLabel=elseif( u1 >= 1.765)
  LUT 1.77RR : Lookup_n-D  NumberOfTableDimensions=1  BreakpointsForDimension1=[408.0552;517.0881;604.0915;696.1871;787.7978;878.8689;969.5172;1059.846;1149.934;1239.836;1329.594;1419.237;1508.789;1598.267;1687.684;1777.05;1866.373]  Table=[400;500;600;700;800;900;1000;1100;1200;1300;1400;1500;1600;1700;1800;1900;2000]  InternalRulePriority=Speed  RndMeth=Simplest
  Out1 : Outport
  wires:
  In1/1 -> LUT 1.77RR/1
  LUT 1.77RR/1 -> Out1/1

== system LUT_kidney_35/If Action Subsystem6/If Action Subsystem2/If Action Subsystem7/If Action Subsystem8 ==
  In1 : Inport
  Action Port : ActionPort  ActionPortLabel=elseif(u1 >= 1.775)
  LUT 1.78RR : Lookup_n-D  NumberOfTableDimensions=1  BreakpointsForDimension1=[407.9471;516.9648;603.9529;696.021;787.5962;878.6257;969.2279;1059.507;1149.543;1239.39;1329.092;1418.678;1508.171;1597.589;1686.946;1776.251;1865.514]  Table=[400;500;600;700;800;900;1000;1100;1200;1300;1400;1500;1600;1700;1800;1900;2000]  InternalRulePriority=Speed  RndMeth=Simplest
  Out1 : Outport
  wires:
  In1/1 -> LUT 1.78RR/1
  LUT 1.78RR/1 -> Out1/1

== system LUT_kidney_35/If Action Subsystem6/If Action Subsystem2/If Action Subsystem7/If Action Subsystem9 ==
  In1 : Inport
  Action Port : ActionPort  ActionPortLabel=if(u1 >= 1.785)
  LUT 1.79RR : Lookup_n-D  NumberOfTableDimensions=1  BreakpointsForDimension1=[407.8399;516.8429;603.8163;695.8577;787.3983;878.3871;968.9439;1059.175;1149.158;1238.952;1328.598;1418.127;1507.563;1596.923;1686.22;1775.466;1864.668]  Table=[400;500;600;700;800;900;1000;1100;1200;1300;1400;1500;1600;1700;1800;1900;2000]  InternalRulePriority=Speed  RndMeth=Simplest
  Out1 : Outport
  wires:
  In1/1 -> LUT 1.79RR/1
  LUT 1.79RR/1 -> Out1/1

== system LUT_kidney_35/If Action Subsystem6/If Action Subsystem2/If Action Subsystem8/If Action Subsystem1 ==
  In1 : Inport
  Action Port : ActionPort  ActionPortLabel=elseif( u1 >= 1.815)
  LUT 1.82RR : Lookup_n-D  NumberOfTableDimensions=1  BreakpointsForDimension1=[407.5242;516.4864;603.4193;695.3847;786.8259;877.6972;968.1227;1058.212;1148.045;1237.683;1327.167;1416.531;1505.799;1594.987;1684.111;1773.181;1862.207]  Table=[400;500;600;700;800;900;1000;1100;1200;1300;1400;1500;1600;1700;1800;1900;2000]  InternalRulePriority=Speed  RndMeth=Simplest
  Out1 : Outport
  wires:
  In1/1 -> LUT 1.82RR/1
  LUT 1.82RR/1 -> Out1/1

== system LUT_kidney_35/If Action Subsystem6/If Action Subsystem2/If Action Subsystem8/If Action Subsystem10 ==
  In1 : Inport
  Action Port : ActionPort  ActionPortLabel=elseif( u1>= 1.805)
  LUT 1.81RR : Lookup_n-D  NumberOfTableDimensions=1  BreakpointsForDimension1=[407.6285;516.6038;603.5496;695.5396;787.0132;877.9229;968.3914;1058.527;1148.409;1238.098;1327.636;1417.054;1506.377;1595.622;1684.803;1773.931;1863.015]  Table=[400;500;600;700;800;900;1000;1100;1200;1300;1400;1500;1600;1700;1800;1900;2000]  InternalRulePriority=Speed  RndMeth=Simplest
  Out1 : Outport
  wires:
  In1/1 -> LUT 1.81RR/1
  LUT 1.81RR/1 -> Out1/1

== system LUT_kidney_35/If Action Subsystem6/If Action Subsystem2/If Action Subsystem8/If Action Subsystem2 ==
  In1 : Inport
  Action Port : ActionPort  ActionPortLabel=else
  LUT 1.80RR : Lookup_n-D  NumberOfTableDimensions=1  BreakpointsForDimension1=[407.7338;516.7226;603.6819;695.6973;787.204;878.1528;968.6651;1058.848;1148.78;1238.521;1328.113;1417.586;1506.965;1596.267;1685.506;1774.692;1863.835]  Table=[400;500;600;700;800;900;1000;1100;1200;1300;1400;1500;1600;1700;1800;1900;2000]  InternalRulePriority=Speed  RndMeth=Simplest
  Out1 : Outport
  wires:
  In1/1 -> LUT 1.80RR/1
  LUT 1.80RR/1 -> Out1/1

== system LUT_kidney_35/If Action Subsystem6/If Action Subsystem2/If Action Subsystem8/If Action Subsystem3 ==
  In1 : Inport
  Action Port : ActionPort  ActionPortLabel=elseif( u1 >= 1.825)
  LUT 1.83RR : Lookup_n-D  NumberOfTableDimensions=1  BreakpointsForDimension1=[407.4208;516.3705;603.2909;695.2324;786.642;877.4757;967.859;1057.902;1147.687;1237.274;1326.707;1416.017;1505.229;1594.362;1683.43;1772.444;1861.412]  Table=[400;500;600;700;800;900;1000;1100;1200;1300;1400;1500;1600;1700;1800;1900;2000]  InternalRulePriority=Speed  RndMeth=Simplest
  Out1 : Outport
  wires:
  In1/1 -> LUT 1.83RR/1
  LUT 1.83RR/1 -> Out1/1

== system LUT_kidney_35/If Action Subsystem6/If Action Subsystem2/If Action Subsystem8/If Action Subsystem4 ==
  In1 : Inport
  Action Port : ActionPort  ActionPortLabel=elseif( u1 >= 1.835)
  LUT 1.84RR : Lookup_n-D  NumberOfTableDimensions=1  BreakpointsForDimension1=[407.3183;516.2559;603.1645;695.0828;786.4615;877.2582;967.6001;1057.598;1147.336;1236.873;1326.254;1415.511;1504.67;1593.748;1682.76;1771.717;1860.629]  Table=[400;500;600;700;800;900;1000;1100;1200;1300;1400;1500;1600;1700;1800;1900;2000]  InternalRulePriority=Speed  RndMeth=Simplest
  Out1 : Outport
  wires:
  In1/1 -> LUT 1.84RR/1
  LUT 1.84RR/1 -> Out1/1

== system LUT_kidney_35/If Action Subsystem6/If Action Subsystem2/If Action Subsystem8/If Action Subsystem5 ==
  In1 : Inport
  Action Port : ActionPort  ActionPortLabel=elseif( u1 >= 1.855)
  LUT 1.86RR : Lookup_n-D  NumberOfTableDimensions=1  BreakpointsForDimension1=[407.116;516.031;602.9173;694.7911;786.1101;876.8353;967.0964;1057.007;1146.651;1236.09;1325.37;1414.524;1503.577;1592.548;1681.451;1770.298;1859.098]  Table=[400;500;600;700;800;900;1000;1100;1200;1300;1400;1500;1600;1700;1800;1900;2000]  InternalRulePriority=Speed  RndMeth=Simplest
  Out1 : Outport
  wires:
  In1/1 -> LUT 1.86RR/1
  LUT 1.86RR/1 -> Out1/1

== system LUT_kidney_35/If Action Subsystem6/If Action Subsystem2/If Action Subsystem8/If Action Subsystem6 ==
  In1 : Inport
  Action Port : ActionPort  ActionPortLabel=elseif( u1 >= 1.845)
  LUT 1.85RR : Lookup_n-D  NumberOfTableDimensions=1  BreakpointsForDimension1=[407.2167;516.1428;603.04;694.9357;786.2842;877.0448;967.3459;1057.3;1146.99;1236.478;1325.808;1415.014;1504.119;1593.143;1682.1;1771.002;1859.858]  Table=[400;500;600;700;800;900;1000;1100;1200;1300;1400;1500;1600;1700;1800;1900;2000]  InternalRulePriority=Speed  RndMeth=Simplest
  Out1 : Outport
  wires:
  In1/1 -> LUT 1.85RR/1
  LUT 1.85RR/1 -> Out1/1

== system LUT_kidney_35/If Action Subsystem6/If Action Subsystem2/If Action Subsystem8/If Action Subsystem7 ==
  In1 : Inport
  Action Port : ActionPort  ActionPortLabel=elseif( u1 >= 1.865)
  LUT 1.87RR : Lookup_n-D  NumberOfTableDimensions=1  BreakpointsForDimension1=[407.0161039;515.9204904;602.7964794;694.649036;785.9392415;876.6296826;966.8514434;1056.718903;1146.317465;1235.709358;1324.940084;1414.043305;1503.044276;1591.962215;1680.811945;1769.605052;1858.350696]  Table=[400;500;600;700;800;900;1000;1100;1200;1300;1400;1500;1600;1700;1800;1900;2000]  InternalRulePriority=Speed  RndMeth=Simplest
  Out1 : Outport
  wires:
  In1/1 -> LUT 1.87RR/1
  LUT 1.87RR/1 -> Out1/1

== system LUT_kidney_35/If Action Subsystem6/If Action Subsystem2/If Action Subsystem8/If Action Subsystem8 ==
  In1 : Inport
  Action Port : ActionPort  ActionPortLabel=elseif(u1 >= 1.875)
  LUT 1.88RR : Lookup_n-D  NumberOfTableDimensions=1  BreakpointsForDimension1=[406.9171;515.8113;602.6775;694.5094;785.7714;876.4278;966.611;1056.436;1145.99;1235.335;1324.517;1413.57;1502.52;1591.386;1680.183;1768.923;1857.614]  Table=[400;500;600;700;800;900;1000;1100;1200;1300;1400;1500;1600;1700;1800;1900;2000]  InternalRulePriority=Speed  RndMeth=Simplest
  Out1 : Outport
  wires:
  In1/1 -> LUT 1.88RR/1
  LUT 1.88RR/1 -> Out1/1

== system LUT_kidney_35/If Action Subsystem6/If Action Subsystem2/If Action Subsystem8/If Action Subsystem9 ==
  In1 : Inport
  Action Port : ActionPort  ActionPortLabel=if(u1 >= 1.885)
  LUT 1.89RR : Lookup_n-D  NumberOfTableDimensions=1  BreakpointsForDimension1=[406.819;515.7035;602.5602;694.3721;785.6067;876.2297;966.375;1056.159;1145.668;1234.967;1324.101;1413.105;1502.004;1590.819;1679.564;1768.251;1856.889]  Table=[400;500;600;700;800;900;1000;1100;1200;1300;1400;1500;1600;1700;1800;1900;2000]  InternalRulePriority=Speed  RndMeth=Simplest
  Out1 : Outport
  wires:
  In1/1 -> LUT 1.89RR/1
  LUT 1.89RR/1 -> Out1/1

== system LUT_kidney_35/If Action Subsystem6/If Action Subsystem2/If Action Subsystem9/If Action Subsystem1 ==
  In1 : Inport
  Action Port : ActionPort  ActionPortLabel=elseif( u1 >= 1.915)
  LUT 1.92RR : Lookup_n-D  NumberOfTableDimensions=1  BreakpointsForDimension1=[406.5296;515.3874;602.2187;693.974;785.1301;875.657;965.6925;1055.356;1144.737;1233.901;1322.895;1411.754;1500.506;1589.171;1677.763;1766.296;1854.779]  Table=[400;500;600;700;800;900;1000;1100;1200;1300;1400;1500;1600;1700;1800;1900;2000]  InternalRulePriority=Speed  RndMeth=Simplest
  Out1 : Outport
  wires:
  In1/1 -> LUT 1.92RR/1
  LUT 1.92RR/1 -> Out1/1

== system LUT_kidney_35/If Action Subsystem6/If Action Subsystem2/If Action Subsystem9/If Action Subsystem10 ==
  In1 : Inport
  Action Port : ActionPort  ActionPortLabel=if(u1 >= 1.995)
  LUT 2.00RR : Lookup_n-D  NumberOfTableDimensions=1  BreakpointsForDimension1=[405.7928;514.5959;601.3779;693.0068;783.9797;874.2777;964.0483;1053.419;1142.485;1231.316;1319.964;1408.466;1496.852;1585.143;1673.356;1761.504;1849.598]  Table=[400;500;600;700;800;900;1000;1100;1200;1300;1400;1500;1600;1700;1800;1900;2000]  InternalRulePriority=Speed  RndMeth=Simplest
  Out1 : Outport
  wires:
  In1/1 -> LUT 2.00RR/1
  LUT 2.00RR/1 -> Out1/1
